simulink model "myo_sfun_one_myo_imu_emg"  (R2019b)
settings: Solver=ode1  StartTime=0.0  StopTime=inf  FixedStep=0.005  RelTol=1e-3  EnableMultiTasking=on
libraries: myo_lib x3, sldrtlib x1
settings Model: Creator=Mark Tomaszewski  LastModifiedBy=bhisma
settings DataIOCC: LimitDataPoints=on  SaveFormat=Array  ReturnWorkspaceOutputs=off
settings OptimizationCC: DefaultParameterBehavior=Inlined  LifeSpan=inf
settings DebuggingCC: UnderspecifiedInitializationDetection=Classic  MergeDetectMultiDrivingBlocksExec=none  SolverPrmCheckMsg=warning  StateNameClashWarn=warning  SFUnexpectedBacktrackingDiag=warning  SFNoUnconditionalDefaultTransitionDiag=warning  SFExecutionAtInitializationDiag=none  ArithmeticOperatorsInVariantConditions=warning
settings HardwareCC: ProdBitPerPointer=32  ProdBitPerSizeT=32  ProdBitPerPtrDiffT=32  ProdLargestAtomicFloat=None  ProdIntDivRoundTo=Undefined  ProdEndianess=Unspecified  ProdWordSize=32  ProdHWDeviceType=32-bit Generic
settings ModelReferenceCC: PropagateSignalLabelsOutOfModel=off
settings SFSimCC: SimUseLocalCustomCode=off  CustomCodeUndefinedFunction=UseInterfaceOnly
settings RTWCC: RTWUseLocalCustomCode=off
settings CodeAppCC: StateflowObjectComments=on
settings GRTTargetCC: TargetLangStandard=C89/C90 (ANSI)  GeneratePreprocessorConditionals=Disable all  ExtMode=on
settings ConfigComp: CovMetricSettings=dw  CovHtmlReporting=on  CovSaveCumulativeToWorkspaceVar=on  CovSaveSingleToWorkspaceVar=on  CovExternalEMLEnable=off

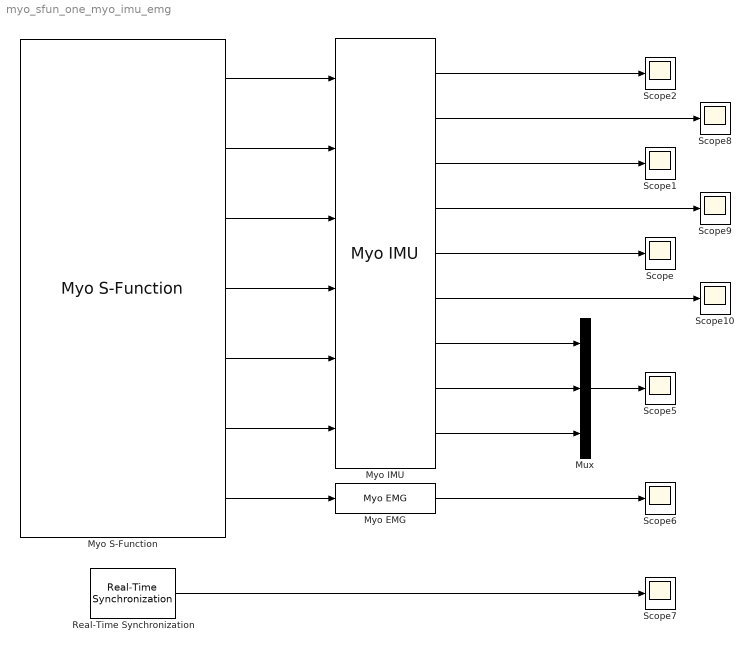
== system myo_sfun_one_myo_imu_emg ==
  Mux : Mux  Inputs=3
  Myo EMG : myo_lib/Myo EMG
  Myo IMU : myo_lib/Myo IMU
  Myo S-Function : myo_lib/Myo S-Function  emgEnabled=1  countMyos=1
  Real-Time Synchronization : sldrtlib/Real-Time Synchronization  SampleTime=0.04  MaxMissedTicks=50  ShowMissedTicks=on  YieldWhenWaiting=on
  Scope{,1..2,5..10} (9 alike) : Scope
  wires:
  Real-Time Synchronization/1 -> Scope7/1
  Mux/1 -> Scope5/1
  Myo S-Function/1 -> Myo IMU/1
  Myo S-Function/2 -> Myo IMU/2
  Myo S-Function/3 -> Myo IMU/3
  Myo S-Function/4 -> Myo IMU/4
  Myo S-Function/5 -> Myo IMU/5
  Myo S-Function/6 -> Myo IMU/6
  Myo S-Function/7 -> Myo EMG/1
  Myo IMU/1 -> Scope2/1
  Myo IMU/2 -> Scope8/1
  Myo IMU/3 -> Scope1/1
  Myo IMU/4 -> Scope9/1
  Myo IMU/5 -> Scope/1
  Myo IMU/6 -> Scope10/1
  Myo IMU/8 -> Mux/2
  Myo IMU/7 -> Mux/1
  Myo IMU/9 -> Mux/3
  Myo EMG/1 -> Scope6/1
